simulink model "Problem5"  (R2020a)
settings: Solver=VariableStepAuto  StartTime=0.0  StopTime=10.0  FixedStep=0.001  RelTol=1e-3
model workspace (MAT data in the model file):
  C = 10
  R = 10
settings Model: OrderedModelArguments=off  Creator=tnradm  LastModifiedBy=tnradm

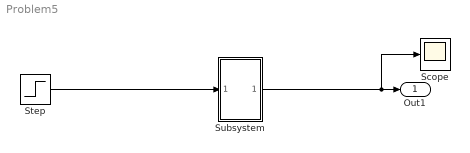
== system Problem5 ==
  Scope : Scope
  Step : Step  SampleTime=0
  Subsystem : Subsystem
  Out1 : Outport
  wires:
  Subsystem/1(Out1) -> Out1/1, Scope/1
  Step/1 -> Subsystem/1(In1)

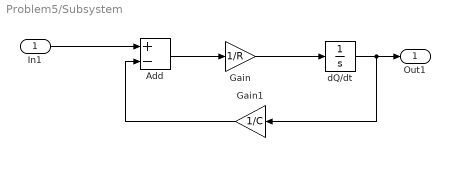
== system Problem5/Subsystem ==
  In1 : Inport
  Add : Sum  Inputs=+-
  Gain : Gain  Gain=1/R  SaturateOnIntegerOverflow=on
  Gain1 : Gain  Gain=1/C  SaturateOnIntegerOverflow=on
  dQ/dt : Integrator
  Out1 : Outport
  wires:
  Gain/1 -> dQ/dt/1
  dQ/dt/1 -> Out1/1, Gain1/1
  Add/1 -> Gain/1
  Gain1/1 -> Add/2
  In1/1 -> Add/1
